simulink model "D53_LKA_Software"  (R2018b)
settings: Solver=ode3  StartTime=0.0  StopTime=10.0  FixedStep=0.01  RelTol=1e-3  EnableMultiTasking=on
model workspace (MAT data in the model file):
  MCOS : class17 (value not decoded)
  MCOS : class17 (value not decoded)
  MCOS : class17 (value not decoded)
  MCOS : class17 (value not decoded)
  MCOS : class17 (value not decoded)
  MCOS : class17 (value not decoded)
  MCOS : class17 (value not decoded)
  MCOS : class17 (value not decoded)
  MCOS : class17 (value not decoded)
  MCOS : class17 (value not decoded)
  MCOS : class17 (value not decoded)
  MCOS : class17 (value not decoded)
  MCOS : class17 (value not decoded)
  MCOS : class17 (value not decoded)
  MCOS : class17 (value not decoded)
  MCOS : class17 (value not decoded)
  MCOS : class17 (value not decoded)
  MCOS : class17 (value not decoded)
  MCOS : class17 (value not decoded)
  MCOS : class17 (value not decoded)
  MCOS : class17 (value not decoded)
  MCOS : class17 (value not decoded)
  MCOS : class17 (value not decoded)
  MCOS : class17 (value not decoded)
  MCOS : class17 (value not decoded)
  MCOS : class17 (value not decoded)
  MCOS : class17 (value not decoded)
  MCOS : class17 (value not decoded)
  MCOS : class17 (value not decoded)
  MCOS : class17 (value not decoded)
  MCOS : class17 (value not decoded)
  MCOS : class17 (value not decoded)
  MCOS : class17 (value not decoded)
  MCOS : class17 (value not decoded)
  MCOS : class17 (value not decoded)
  MCOS : class17 (value not decoded)
  MCOS : class17 (value not decoded)
  MCOS : class17 (value not decoded)
  MCOS : class17 (value not decoded)
  MCOS : class17 (value not decoded)
  MCOS : class17 (value not decoded)
  MCOS : class17 (value not decoded)
  MCOS : class17 (value not decoded)
  MCOS : class17 (value not decoded)
  MCOS : class17 (value not decoded)
  MCOS : class17 (value not decoded)
  MCOS : class17 (value not decoded)
  MCOS : class17 (value not decoded)
  MCOS : class17 (value not decoded)
  MCOS : class17 (value not decoded)
  MCOS : class17 (value not decoded)
  MCOS : class17 (value not decoded)
  MCOS : class17 (value not decoded)
  MCOS : class17 (value not decoded)
  MCOS : class17 (value not decoded)
  MCOS : class17 (value not decoded)
  MCOS : class17 (value not decoded)
  MCOS : class17 (value not decoded)
  MCOS : class17 (value not decoded)
  MCOS : class17 (value not decoded)
  MCOS : class17 (value not decoded)
  MCOS : class17 (value not decoded)
  MCOS : class17 (value not decoded)
  MCOS : class17 (value not decoded)
  MCOS : class17 (value not decoded)
  MCOS : class17 (value not decoded)
  MCOS : class17 (value not decoded)
  MCOS : class17 (value not decoded)
  MCOS : class17 (value not decoded)
  MCOS : class17 (value not decoded)
  MCOS : class17 (value not decoded)
  MCOS : class17 (value not decoded)
  MCOS : class17 (value not decoded)
  MCOS : class17 (value not decoded)
  MCOS : class17 (value not decoded)
  MCOS : class17 (value not decoded)
  MCOS : class17 (value not decoded)
  MCOS : class17 (value not decoded)
  MCOS : class17 (value not decoded)
  MCOS : class17 (value not decoded)
  MCOS : class17 (value not decoded)
  MCOS : class17 (value not decoded)
  MCOS : class17 (value not decoded)
  MCOS : class17 (value not decoded)
  MCOS : class17 (value not decoded)
  MCOS : class17 (value not decoded)
  MCOS : class17 (value not decoded)
  MCOS : class17 (value not decoded)
  MCOS : class17 (value not decoded)
undefined symbols (not defined in the file or in its folder): LKA_CarWidth, LKA_SampleTime, LKA_StrRatio_C, LKA_Veh2CamL_C, LKA_Veh2CamW_C, LKA_WhlBaseL_C, LL_CompSWA_C, LL_CrvtPrvwT_C, LL_DesDvt_C, LL_DvtComp_C, LL_DvtPrvwT_C, LL_DvtSpdDet_vDvtSpdMin_C, LL_HdAgExT_C, LL_HdAgPrvwT_C, LL_LAccMax_C, LL_LAccRMax_C, LL_LDW_EarliestWarnLine_C, LL_LDW_LatestWarnLine_C, LL_LDWS_SUPPRESS_HEADING, LL_LFClb_TFC_DiffCtlBalance, LL_LFClb_TFC_DiffCtrlMaxSWA, LL_LFClb_TFC_DiffCtrlRatio, LL_LFClb_TFC_facmGainLutGain1_C, LL_LFClb_TFC_facmGainLutGain2_C, LL_LFClb_TFC_facmIntegRatio, LL_LFClb_TFC_facmKlat_C, LL_LFClb_TFC_FfCtlRatio_C, LL_LFClb_TFC_phiIntegCtlMaxSWA_C, LL_LFClb_TFC_tiKlatPrvwT_C, LL_LFClb_TFC_vGainLutVehSpdLwr_C, LL_LFClb_TFC_vGainLutVehSpdUpr_C, LL_LKA_EarliestWarnLine_C, LL_LKA_LatestWarnLine_C, LL_LKAExPrcs_ExitC0Dvt, LL_LKAExPrcs_ExitC0Swt, LL_LKAExPrcs_tiExitTime1, LL_LKAExPrcs_tiExitTime2, LL_LKAExPrcs_tiExitTime3, LL_LKAS_OUT_OF_CONTROL_LAT_VEL, LL_LKAS_OUT_OF_CONTROL_TTLC, LL_LKASWASyn_M0, LL_LKASWASyn_M1, LL_LKASWASyn_M2, LL_LKASWASyn_M3K, LL_LKASWASyn_SWAaddMax, LL_LKASWASyn_T2, LL_LKASWASyn_tiTrqSwaRtTime, LL_LKASWASyn_tiTrqSwaTime, LL_LKASWASyn_TrqMax, LL_LKASWASyn_TrqSwaAddSwt, LL_LKASWASyn_TrqSwaRateDiff, LL_LSpdCompT_C, LL_lStpLngth_C, LL_MAX_DELAY_EPSSTAR_TIME, LL_MAX_DRIVER_TORQUE_DISABLE, LL_MAX_DRIVER_TORQUE_ENABLE, LL_MAX_LANE_WIDTH_DISABLE, LL_MAX_LANE_WIDTH_ENABLE, LL_MAX_LAT_ACC_DISABLE, LL_MAX_LAT_ACC_ENABLE ... (+30)
libraries: simulink x167, canmsglib x52, dspstat3 x3, simulink_extras x1
(part 5 of 21)

== system D53_LKA_Software/LLClb_bsLLClb_Read_Num=100/Subsystem2 ==
  In1 : Inport
  In2 : Inport  Port=2
  Data Type Conversion{1..10} (10 alike) : DataTypeConversion  OutDataTypeStr=single
  If1 : If  IfExpression=u1 ==1  ElseIfExpressions=u1==2,u1==3,u1==4,u1==5,u1==6,u1==7,u1==8,u1==9,u1==10  ShowElse=off
  Rate Transition{1..3,5..11} (10 alike) : RateTransition  Deterministic=off  OutPortSampleTime=0.01
  Subsystem2 : Subsystem
  Out1 : Outport
  Out2 : Outport  Port=2
  Out3 : Outport  Port=3
  Out4 : Outport  Port=4
  Out5 : Outport  Port=5
  Out6 : Outport  Port=6
  Out7 : Outport  Port=7
  Out8 : Outport  Port=8
  Out9 : Outport  Port=9
  Out10 : Outport  Port=10
  wires:
  Subsystem2/10(Out10) -> Data Type Conversion10/1
  Subsystem2/4(Out4) -> Data Type Conversion4/1
  If1/3 -> Subsystem2/3(In3)
  Subsystem2/7(Out7) -> Data Type Conversion7/1
  Subsystem2/1(Out1) -> Data Type Conversion1/1
  Subsystem2/9(Out9) -> Data Type Conversion9/1
  If1/6 -> Subsystem2/6(In6)
  If1/2 -> Subsystem2/2(In2)
  If1/5 -> Subsystem2/5(In5)
  Subsystem2/8(Out8) -> Data Type Conversion8/1
  If1/9 -> Subsystem2/9(In9)
  If1/4 -> Subsystem2/4(In4)
  If1/1 -> Subsystem2/1(In1)
  If1/7 -> Subsystem2/7(In7)
  If1/8 -> Subsystem2/8(In8)
  Subsystem2/3(Out3) -> Data Type Conversion3/1
  Subsystem2/2(Out2) -> Data Type Conversion2/1
  If1/10 -> Subsystem2/10(In10)
  Subsystem2/5(Out5) -> Data Type Conversion5/1
  Subsystem2/6(Out6) -> Data Type Conversion6/1
  In1/1 -> If1/1
  In2/1 -> Subsystem2/11(In11)
  Data Type Conversion1/1 -> Rate Transition1/1
  Data Type Conversion2/1 -> Rate Transition2/1
  Data Type Conversion3/1 -> Rate Transition3/1
  Data Type Conversion4/1 -> Rate Transition5/1
  Data Type Conversion5/1 -> Rate Transition6/1
  Data Type Conversion6/1 -> Rate Transition7/1
  Data Type Conversion7/1 -> Rate Transition8/1
  Data Type Conversion8/1 -> Rate Transition9/1
  Data Type Conversion9/1 -> Rate Transition10/1
  Data Type Conversion10/1 -> Rate Transition11/1
  Rate Transition1/1 -> Out1/1
  Rate Transition2/1 -> Out2/1
  Rate Transition3/1 -> Out3/1
  Rate Transition5/1 -> Out4/1
  Rate Transition6/1 -> Out5/1
  Rate Transition7/1 -> Out6/1
  Rate Transition8/1 -> Out7/1
  Rate Transition9/1 -> Out8/1
  Rate Transition10/1 -> Out9/1
  Rate Transition11/1 -> Out10/1

== system D53_LKA_Software/LLClb_bsLLClb_Read_Num=100/Subsystem3 ==
  In1 : Inport
  In2 : Inport  Port=2
  Data Type Conversion{1..10} (10 alike) : DataTypeConversion  OutDataTypeStr=single
  If1 : If  IfExpression=u1 ==11  ElseIfExpressions=u1==12,u1==13,u1==14,u1==15,u1==16,u1==17,u1==18,u1==19,u1==20  ShowElse=off
  Rate Transition{1..3,5..11} (10 alike) : RateTransition  Deterministic=off  OutPortSampleTime=0.01
  Subsystem2 : Subsystem
  Out1 : Outport
  Out2 : Outport  Port=2
  Out3 : Outport  Port=3
  Out4 : Outport  Port=4
  Out5 : Outport  Port=5
  Out6 : Outport  Port=6
  Out7 : Outport  Port=7
  Out8 : Outport  Port=8
  Out9 : Outport  Port=9
  Out10 : Outport  Port=10
  wires:
  If1/10 -> Subsystem2/10(In10)
  If1/8 -> Subsystem2/8(In8)
  If1/7 -> Subsystem2/7(In7)
  If1/1 -> Subsystem2/1(In1)
  If1/4 -> Subsystem2/4(In4)
  If1/9 -> Subsystem2/9(In9)
  If1/5 -> Subsystem2/5(In5)
  If1/2 -> Subsystem2/2(In2)
  If1/6 -> Subsystem2/6(In6)
  If1/3 -> Subsystem2/3(In3)
  In2/1 -> Subsystem2/11(In11)
  In1/1 -> If1/1
  Data Type Conversion3/1 -> Rate Transition3/1
  Data Type Conversion2/1 -> Rate Transition2/1
  Data Type Conversion10/1 -> Rate Transition11/1
  Data Type Conversion5/1 -> Rate Transition6/1
  Rate Transition6/1 -> Out5/1
  Subsystem2/5(Out5) -> Data Type Conversion5/1
  Subsystem2/6(Out6) -> Data Type Conversion6/1
  Subsystem2/10(Out10) -> Data Type Conversion10/1
  Subsystem2/1(Out1) -> Data Type Conversion1/1
  Subsystem2/9(Out9) -> Data Type Conversion9/1
  Subsystem2/7(Out7) -> Data Type Conversion7/1
  Subsystem2/8(Out8) -> Data Type Conversion8/1
  Subsystem2/3(Out3) -> Data Type Conversion3/1
  Subsystem2/4(Out4) -> Data Type Conversion4/1
  Data Type Conversion4/1 -> Rate Transition5/1
  Data Type Conversion8/1 -> Rate Transition9/1
  Data Type Conversion9/1 -> Rate Transition10/1
  Data Type Conversion7/1 -> Rate Transition8/1
  Rate Transition8/1 -> Out7/1
  Rate Transition1/1 -> Out1/1
  Rate Transition2/1 -> Out2/1
  Rate Transition5/1 -> Out4/1
  Rate Transition10/1 -> Out9/1
  Rate Transition11/1 -> Out10/1
  Rate Transition3/1 -> Out3/1
  Subsystem2/2(Out2) -> Data Type Conversion2/1
  Data Type Conversion6/1 -> Rate Transition7/1
  Rate Transition7/1 -> Out6/1
  Data Type Conversion1/1 -> Rate Transition1/1
  Rate Transition9/1 -> Out8/1

== system D53_LKA_Software/LLClb_bsLLClb_Read_Num=100/Subsystem4 ==
  In1 : Inport
  In2 : Inport  Port=2
  Data Type Conversion{1..10} (10 alike) : DataTypeConversion  OutDataTypeStr=single
  If1 : If  IfExpression=u1 ==21  ElseIfExpressions=u1==22,u1==23,u1==24,u1==25,u1==26,u1==27,u1==28,u1==29,u1==30  ShowElse=off
  Rate Transition{1..3,5..11} (10 alike) : RateTransition  Deterministic=off  OutPortSampleTime=0.01
  Subsystem2 : Subsystem
  Out1 : Outport
  Out2 : Outport  Port=2
  Out3 : Outport  Port=3
  Out4 : Outport  Port=4
  Out5 : Outport  Port=5
  Out6 : Outport  Port=6
  Out7 : Outport  Port=7
  Out8 : Outport  Port=8
  Out9 : Outport  Port=9
  Out10 : Outport  Port=10
  wires:
  If1/3 -> Subsystem2/3(In3)
  If1/6 -> Subsystem2/6(In6)
  If1/2 -> Subsystem2/2(In2)
  If1/5 -> Subsystem2/5(In5)
  If1/9 -> Subsystem2/9(In9)
  If1/4 -> Subsystem2/4(In4)
  If1/1 -> Subsystem2/1(In1)
  If1/7 -> Subsystem2/7(In7)
  If1/8 -> Subsystem2/8(In8)
  If1/10 -> Subsystem2/10(In10)
  In1/1 -> If1/1
  In2/1 -> Subsystem2/11(In11)
  Data Type Conversion3/1 -> Rate Transition3/1
  Data Type Conversion2/1 -> Rate Transition2/1
  Data Type Conversion10/1 -> Rate Transition11/1
  Data Type Conversion5/1 -> Rate Transition6/1
  Rate Transition6/1 -> Out5/1
  Subsystem2/5(Out5) -> Data Type Conversion5/1
  Subsystem2/6(Out6) -> Data Type Conversion6/1
  Subsystem2/10(Out10) -> Data Type Conversion10/1
  Subsystem2/1(Out1) -> Data Type Conversion1/1
  Subsystem2/9(Out9) -> Data Type Conversion9/1
  Subsystem2/7(Out7) -> Data Type Conversion7/1
  Subsystem2/8(Out8) -> Data Type Conversion8/1
  Subsystem2/3(Out3) -> Data Type Conversion3/1
  Subsystem2/4(Out4) -> Data Type Conversion4/1
  Data Type Conversion4/1 -> Rate Transition5/1
  Data Type Conversion8/1 -> Rate Transition9/1
  Data Type Conversion9/1 -> Rate Transition10/1
  Data Type Conversion7/1 -> Rate Transition8/1
  Rate Transition8/1 -> Out7/1
  Rate Transition1/1 -> Out1/1
  Rate Transition2/1 -> Out2/1
  Rate Transition5/1 -> Out4/1
  Rate Transition10/1 -> Out9/1
  Rate Transition11/1 -> Out10/1
  Rate Transition3/1 -> Out3/1
  Subsystem2/2(Out2) -> Data Type Conversion2/1
  Data Type Conversion6/1 -> Rate Transition7/1
  Rate Transition7/1 -> Out6/1
  Data Type Conversion1/1 -> Rate Transition1/1
  Rate Transition9/1 -> Out8/1

== system D53_LKA_Software/LLClb_bsLLClb_Read_Num=100/Subsystem5 ==
  In1 : Inport
  In2 : Inport  Port=2
  Constant : Constant  Value=10
  Data Type Conversion1 : DataTypeConversion  OutDataTypeStr=single
  Data Type Conversion3 : DataTypeConversion  OutDataTypeStr=single
  Divide : Product  Inputs=**
  Fcn : Fcn  Expr=pow(u(1),u(2))
  Mux : Mux  Inputs=2
  Out1 : Outport
  wires:
  Mux/1 -> Fcn/1
  Fcn/1 -> Divide/1
  In2/1 -> Divide/2
  Divide/1 -> Out1/1
  In1/1 -> Data Type Conversion1/1
  Data Type Conversion1/1 -> Mux/2
  Data Type Conversion3/1 -> Mux/1
  Constant/1 -> Data Type Conversion3/1

== system D53_LKA_Software/Resource Initialization/CAN Setup ==
  S-Function : S-Function  FunctionName=CAN_Init_D  Parameters=uint8(Device_Index-1),uint8(CAN0_En),uint8(CAN0_Baudrate-1),uint8(CAN1_En),uint8(CAN1_Baudrate-1),uint8(CAN2_En),uint8(CAN2_Baudrate-1),uint8(CAN3_En),uint8(CAN3_Baudrate-1)  SFunctionDeploymentMode=off  EnableBusSupport=off

== system D53_LKA_Software/Resource Initialization/DI ==

== system D53_LKA_Software/Resource Initialization/DO ==

== system D53_LKA_Software/Resource Initialization/SPI ==

== system D53_LKA_Software/Signal Output and Processing (DACOut)/D53_EPS_Control_LKA ==
  LKA_STATE_in : Inport
  LXA_ACTIVATION_in : Inport  Port=2
  LKA_TRQ_FACT_REQ_in : Inport  Port=3
  COLUMN_ANGLE_SETPOINT_in : Inport  Port=4
  Constant{2..9} (8 alike) : Constant  Value=0  OutDataTypeStr=single
  Data Type Conversion : DataTypeConversion  OutDataTypeStr=single
  DMD_DELEST_ABS_ESP : Outport
  REQ_DECON_ASR : Outport  Port=2
  LKA_TRQ_FACT_REQ : Outport  Port=3
  COLUMN_ANGLE_SETPOINT : Outport  Port=4
  ACPK_VAL_REQUEST_BSI : Outport  Port=5
  DMD_DELEST_EASYMOVE : Outport  Port=6
  LKA_STATE : Outport  Port=7
  LXA_ACTIVATION : Outport  Port=8
  DMD_DELEST_DA : Outport  Port=9
  TRAILER_DETECTION : Outport  Port=10
  CPT_PROCESS : Outport  Port=11
  CHKSUM_TRME : Outport  Port=12
  wires:
  LKA_STATE_in/1 -> Data Type Conversion/1
  Data Type Conversion/1 -> LKA_STATE/1
  COLUMN_ANGLE_SETPOINT_in/1 -> COLUMN_ANGLE_SETPOINT/1
  Constant2/1 -> DMD_DELEST_DA/1
  LXA_ACTIVATION_in/1 -> LXA_ACTIVATION/1
  LKA_TRQ_FACT_REQ_in/1 -> LKA_TRQ_FACT_REQ/1
  Constant3/1 -> TRAILER_DETECTION/1
  Constant4/1 -> DMD_DELEST_EASYMOVE/1
  Constant5/1 -> DMD_DELEST_ABS_ESP/1
  Constant6/1 -> CHKSUM_TRME/1
  Constant7/1 -> CPT_PROCESS/1
  Constant8/1 -> REQ_DECON_ASR/1
  Constant9/1 -> ACPK_VAL_REQUEST_BSI/1

== system D53_LKA_Software/Signal Output and Processing (DACOut)/D53_HMI_Control_LKA ==
  LL_bsLLHMI : Inport
  Bus Selector3 : BusSelector  OutputSignals=Hands_off_warning,HMI_Popup_Status,LDW_Flag,LDW_Status_Display,LKA_action_indication,LKA_Status_Display,Vehicle_Lane_Display
  Constant{,1..7} (8 alike) : Constant  Value=0  OutDataTypeStr=uint16
  ECU_operating_phase : Outport
  HMI_Popup_Status : Outport  Port=2
  Hands_off_warning : Outport  Port=3
  ISA_Popup_text : Outport  Port=4
  ISA_Sign_Type : Outport  Port=5
  ISA_Status : Outport  Port=6
  ISA_Value : Outport  Port=7
  LDW_Flag : Outport  Port=8
  LDW_Status_Display : Outport  Port=9
  LKA_Mode_from_Camera : Outport  Port=10
  LKA_Status_Display : Outport  Port=11
  LKA_Switch_State : Outport  Port=12
  LKA_action_indication : Outport  Port=13
  TSR_Vision_Only_Sign_Type : Outport  Port=14
  Vehicle_Lane_Display : Outport  Port=15
  wires:
  Bus Selector3/1 -> Hands_off_warning/1  "<Hands_off_warning>"
  Bus Selector3/3 -> LDW_Flag/1  "<LDW_Flag>"
  Bus Selector3/4 -> LDW_Status_Display/1  "<LDW_Status_Display>"
  Bus Selector3/5 -> LKA_action_indication/1  "<LKA_action_indication>"
  Bus Selector3/6 -> LKA_Status_Display/1  "<LKA_Status_Display>"
  Bus Selector3/7 -> Vehicle_Lane_Display/1  "<Vehicle_Lane_Display>"
  Bus Selector3/2 -> HMI_Popup_Status/1  "<HMI_Popup_Status>"
  LL_bsLLHMI/1 -> Bus Selector3/1
  Constant/1 -> ECU_operating_phase/1
  Constant1/1 -> ISA_Popup_text/1
  Constant2/1 -> ISA_Sign_Type/1
  Constant4/1 -> ISA_Value/1
  Constant3/1 -> ISA_Status/1
  Constant5/1 -> LKA_Mode_from_Camera/1
  Constant6/1 -> LKA_Switch_State/1
  Constant7/1 -> TSR_Vision_Only_Sign_Type/1

== system D53_LKA_Software/SignalBusCreator/Body Electric System State Receive and Processing (BESRx) ==
  Bus Creator1 : BusCreator  Inputs=11
  Steering Lamp CAN Frame PreProcess (StLampCANFrmPPrcs) : Subsystem
  bsDoorsState : Constant  Value=0  OutDataTypeStr=uint16
  bsWiperState : Constant  Value=0  OutDataTypeStr=uint16
  BESRx_bsBESState : Outport
  wires:
  Steering Lamp CAN Frame PreProcess (StLampCANFrmPPrcs)/9(Out9) -> Bus Creator1/11  "MP5_AEB_Activation_Config"
  bsWiperState/1 -> Bus Creator1/3  "bsWiperState"
  bsDoorsState/1 -> Bus Creator1/2  "bsDoorsState"
  Bus Creator1/1 -> BESRx_bsBESState/1
  Steering Lamp CAN Frame PreProcess (StLampCANFrmPPrcs)/6(Out6) -> Bus Creator1/8  "IC_FCW_Sensitivity"
  Steering Lamp CAN Frame PreProcess (StLampCANFrmPPrcs)/5(Out5) -> Bus Creator1/7  "GW_BCM_Brakeonly_Request_BCM"
  Steering Lamp CAN Frame PreProcess (StLampCANFrmPPrcs)/3(Out3) -> Bus Creator1/6  "BCM_State_Front_Wiper"
  Steering Lamp CAN Frame PreProcess (StLampCANFrmPPrcs)/2(Out2) -> Bus Creator1/5  "BCM_CHMSLStatus"
  Steering Lamp CAN Frame PreProcess (StLampCANFrmPPrcs)/1(Out1) -> Bus Creator1/4  "BCM_BrakeLampStatu"
  Steering Lamp CAN Frame PreProcess (StLampCANFrmPPrcs)/4(CANFrmPPrcs_stLStLamp) -> Bus Creator1/1  "StrLampRx_bsStrLampState"
  Steering Lamp CAN Frame PreProcess (StLampCANFrmPPrcs)/7(Out7) -> Bus Creator1/9  "IC_Fcw_Activation_Config"
  Steering Lamp CAN Frame PreProcess (StLampCANFrmPPrcs)/8(Out8) -> Bus Creator1/10  "IC_seat_bealt_passenger_state"

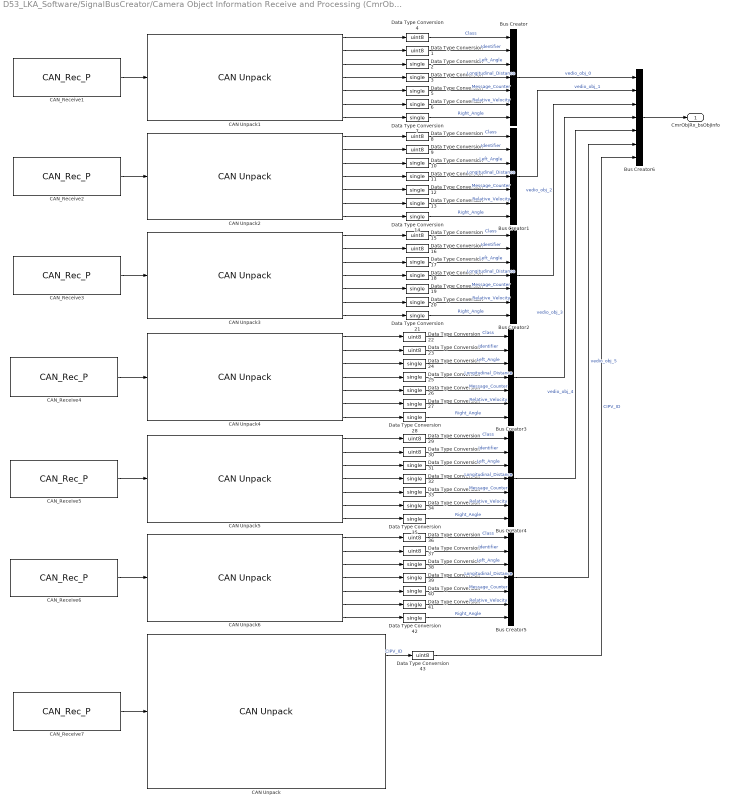
== system D53_LKA_Software/SignalBusCreator/Camera Object Information Receive and Processing (CmrObjRx) ==
  Bus Creator{,1..6} (7 alike) : BusCreator  Inputs=7
  CAN Unpack : canmsglib/CAN Unpack  CANdbFile=F:\ADAS_File\ACC_AEB_D53_20190520\ADAS_ECU_S_CAN_V2_v20190314.dbc  MsgList=Video_Object_Header  MsgName=Video_Object_Header  MsgIDType=Standard (11-bit identifier)  MsgIdentifier=1078  MsgLength=6  SignalInfo=AEB_Availability$0$1$2$2$1$0$1$0$0$1$#CIPV_FCV$9$2$2$2$1$0$1$0$0$3$#CIPV_ID$25$7$2$2$1$0$1$0$0$127$#Left_Close_Range_Cut_In$2$1$2$2$1$0$1$0$0$1$#MCPB_FCV$46$2$2$2$1$0$1$0$0$3$#MCPB_ID$33$7$2$2$1$0$1$0$0$127$#Message_Counter$22$2$2$2$1$0$1$0$0$3$#Number_Of_Objects$3$5$2$2$1$0$1$0$0$31$#PED_CYC_ABA_ALERT$17$1$2$2$1$0$1$0$0$1$#PED_CYC_AEB_ALERT$16$1$2$2$1$0$1$0$0$1$#PED_CYC_DANGER_ZONE$20$2$2$2$1$0$1$0$0$3$#PED_CYC_FCW_ALERT$19$1$2$2$1$0$1$0$0$1$#PED_CYC_PREFILL_ALERT$18$1$2$2$1$0$1$0$0$1$#Right_Close_Range_Cut_In$1$1$2$2$1$0$1$0$0$1$#VEH_ABA_ALERT$13$1$2$2$1$0$1$0$0$1$#VEH_AEB_ALERT$12$1$2$2$1$0$1$0$0$1$#VEH_FCW_ALERT$15$1$2$2$1$0$1$0$0$1$#VEH_PREFILL_ALERT$14$1$2$2$1$0$1$0$0$1$#VEH_RESERVED_ALERT$11$1$2$2$1$0$1$0$0$1$#  NSignals=19  IDPort=off  TimestampPort=off  ErrorPort=off  RemotePort=off  LengthPort=off  StatusPort=off  StartBits=str2num('[int32(0);int32(9);int32(25);int32(2);int32(46);int32(33);int32(22);int32(3);int32(17);int32(16);int32(20);int32(19);int32(18);int32(1);int32(13);int32(12);int32(15);int32(14);int32(11)]')  SignalSizes=str2num('[int32(1);int32(2);int32(7);int32(1);int32(2);int32(7);int32(2);int32(5);int32(1);int32(1);int32(2);int32(1);int32(1);int32(1);int32(1);int32(1);int32(1);int32(1);int32(1)]')  ByteOrders=str2num('[int32(2);int32(2);int32(2);int32(2);int32(2);int32(2);int32(2);int32(2);int32(2);int32(2);int32(2);int32(2);int32(2);int32(2);int32(2);int32(2);int32(2);int32(2);int32(2)]')  DataTypes=str2num('[int32(2);int32(2);int32(2);int32(2);int32(2);int32(2);int32(2);int32(2);int32(2);int32(2);int32(2);int32(2);int32(2);int32(2);int32(2);int32(2);int32(2);int32(2);int32(2)]')  MultiplexTypes=str2num('[int32(1);int32(1);int32(1);int32(1);int32(1);int32(1);int32(1);int32(1);int32(1);int32(1);int32(1);int32(1);int32(1);int32(1);int32(1);int32(1);int32(1);int32(1);int32(1)]')  MultiplexValues=str2num('[double(0);double(0);double(0);double(0);double(0);double(0);double(0);double(0);double(0);double(0);double(0);double(0);double(0);double(0);double(0);double(0);double(0);double(0);double(0)]')  Factors=str2num('[double(1);double(1);double(1);double(1);double(1);double(1);double(1);double(1);double(1);double(1);double(1);double(1);double(1);double(1);double(1);double(1);double(1);double(1);double(1)]')  Offsets=str2num('[double(0);double(0);double(0);double(0);double(0);double(0);double(0);double(0);double(0);double(0);double(0);double(0);double(0);double(0);double(0);double(0);double(0);double(0);double(0)]')  Minimums=str2num('[double(0);double(0);double(0);double(0);double(0);double(0);double(0);double(0);double(0);double(0);double(0);double(0);double(0);double(0);double(0);double(0);double(0);double(0);double(0)]')  Maximums=str2num('[double(1);double(3);double(127);double(1);double(3);double(127);double(3);double(31);double(1);double(1);double(3);double(1);double(1);double(1);double(1);double(1);double(1);double(1);double(1)]')  ApplyMinMax=off
      settings: SourceProductName=Simulink Real-Time  SourceProductBaseCode=XP  DataFormat=CANdb specified signals
  CAN Unpack1 : canmsglib/CAN Unpack  CANdbFile=F:\ADAS_File\ACC_AEB_D53_20190520\ADAS_ECU_S_CAN_V2_v20190314.dbc  MsgList=Video_Object_0_A  MsgName=Video_Object_0_A  MsgIDType=Standard (11-bit identifier)  MsgIdentifier=1792  MsgLength=8  SignalInfo=Class_700$56$3$2$2$1$0$1$0$0$7$#Identifier_700$1$7$2$2$1$0$1$0$0$127$#Left_Angle_700$41$13$2$1$1$0$2.000000e-04$0$-8.192000e-01$8.190000e-01$#Longitudinal_Distance_700$20$12$2$2$1$0$5.000000e-02$0$0$2.047500e+02$#Message_Counter_700$38$2$2$2$1$0$1$0$0$3$#Relative_Velocity_700$24$12$2$1$1$0$5.000000e-02$0$-1.024000e+02$1.023500e+02$#Right_Angle_700$59$13$2$1$1$0$2.000000e-04$0$-8.192000e-01$8.190000e-01$#  NSignals=7  IDPort=off  TimestampPort=off  ErrorPort=off  RemotePort=off  LengthPort=off  StatusPort=off  StartBits=str2num('[int32(56);int32(1);int32(41);int32(20);int32(38);int32(24);int32(59)]')  SignalSizes=str2num('[int32(3);int32(7);int32(13);int32(12);int32(2);int32(12);int32(13)]')  ByteOrders=str2num('[int32(2);int32(2);int32(2);int32(2);int32(2);int32(2);int32(2)]')  DataTypes=str2num('[int32(2);int32(2);int32(1);int32(2);int32(2);int32(1);int32(1)]')  MultiplexTypes=str2num('[int32(1);int32(1);int32(1);int32(1);int32(1);int32(1);int32(1)]')  MultiplexValues=str2num('[double(0);double(0);double(0);double(0);double(0);double(0);double(0)]')  Factors=str2num('[double(1);double(1);double(2.000000e-04);double(5.000000e-02);double(1);double(5.000000e-02);double(2.000000e-04)]')  Offsets=str2num('[double(0);double(0);double(0);double(0);double(0);double(0);double(0)]')  Minimums=str2num('[double(0);double(0);double(-8.192000e-01);double(0);double(0);double(-1.024000e+02);double(-8.192000e-01)]')  Maximums=str2num('[double(7);double(127);double(8.190000e-01);double(2.047500e+02);double(3);double(1.023500e+02);double(8.190000e-01)]')  ApplyMinMax=off
      settings: SourceProductName=Simulink Real-Time  SourceProductBaseCode=XP  DataFormat=CANdb specified signals
  CAN Unpack2 : canmsglib/CAN Unpack  CANdbFile=F:\ADAS_File\ACC_AEB_D53_20190520\ADAS_ECU_S_CAN_V2_v20190314.dbc  MsgList=Video_Object_1_A  MsgName=Video_Object_1_A  MsgIDType=Standard (11-bit identifier)  MsgIdentifier=1796  MsgLength=8  SignalInfo=Class_704$56$3$2$2$1$0$1$0$0$7$#Identifier_704$1$7$2$2$1$0$1$0$0$127$#Left_Angle_704$41$13$2$1$1$0$2.000000e-04$0$-8.192000e-01$8.190000e-01$#Longitudinal_Distance_704$20$12$2$2$1$0$5.000000e-02$0$0$2.047500e+02$#Message_Counter_704$38$2$2$2$1$0$1$0$0$3$#Relative_Velocity_704$24$12$2$1$1$0$5.000000e-02$0$-1.024000e+02$1.023500e+02$#Right_Angle_704$59$13$2$1$1$0$2.000000e-04$0$-8.192000e-01$8.190000e-01$#  NSignals=7  IDPort=off  TimestampPort=off  ErrorPort=off  RemotePort=off  LengthPort=off  StatusPort=off  StartBits=str2num('[int32(56);int32(1);int32(41);int32(20);int32(38);int32(24);int32(59)]')  SignalSizes=str2num('[int32(3);int32(7);int32(13);int32(12);int32(2);int32(12);int32(13)]')  ByteOrders=str2num('[int32(2);int32(2);int32(2);int32(2);int32(2);int32(2);int32(2)]')  DataTypes=str2num('[int32(2);int32(2);int32(1);int32(2);int32(2);int32(1);int32(1)]')  MultiplexTypes=str2num('[int32(1);int32(1);int32(1);int32(1);int32(1);int32(1);int32(1)]')  MultiplexValues=str2num('[double(0);double(0);double(0);double(0);double(0);double(0);double(0)]')  Factors=str2num('[double(1);double(1);double(2.000000e-04);double(5.000000e-02);double(1);double(5.000000e-02);double(2.000000e-04)]')  Offsets=str2num('[double(0);double(0);double(0);double(0);double(0);double(0);double(0)]')  Minimums=str2num('[double(0);double(0);double(-8.192000e-01);double(0);double(0);double(-1.024000e+02);double(-8.192000e-01)]')  Maximums=str2num('[double(7);double(127);double(8.190000e-01);double(2.047500e+02);double(3);double(1.023500e+02);double(8.190000e-01)]')  ApplyMinMax=off
      settings: SourceProductName=Simulink Real-Time  SourceProductBaseCode=XP  DataFormat=CANdb specified signals
  CAN Unpack3 : canmsglib/CAN Unpack  CANdbFile=F:\ADAS_File\ACC_AEB_D53_20190520\ADAS_ECU_S_CAN_V2_v20190314.dbc  MsgList=Video_Object_2_A  MsgName=Video_Object_2_A  MsgIDType=Standard (11-bit identifier)  MsgIdentifier=1800  MsgLength=8  SignalInfo=Class_708$56$3$2$2$1$0$1$0$0$7$#Identifier_708$1$7$2$2$1$0$1$0$0$127$#Left_Angle_708$41$13$2$1$1$0$2.000000e-04$0$-8.192000e-01$8.190000e-01$#Longitudinal_Distance_708$20$12$2$2$1$0$5.000000e-02$0$0$2.047500e+02$#Message_Counter_708$38$2$2$2$1$0$1$0$0$3$#Relative_Velocity_708$24$12$2$1$1$0$5.000000e-02$0$-1.024000e+02$1.023500e+02$#Right_Angle_708$59$13$2$1$1$0$2.000000e-04$0$-8.192000e-01$8.190000e-01$#  NSignals=7  IDPort=off  TimestampPort=off  ErrorPort=off  RemotePort=off  LengthPort=off  StatusPort=off  StartBits=str2num('[int32(56);int32(1);int32(41);int32(20);int32(38);int32(24);int32(59)]')  SignalSizes=str2num('[int32(3);int32(7);int32(13);int32(12);int32(2);int32(12);int32(13)]')  ByteOrders=str2num('[int32(2);int32(2);int32(2);int32(2);int32(2);int32(2);int32(2)]')  DataTypes=str2num('[int32(2);int32(2);int32(1);int32(2);int32(2);int32(1);int32(1)]')  MultiplexTypes=str2num('[int32(1);int32(1);int32(1);int32(1);int32(1);int32(1);int32(1)]')  MultiplexValues=str2num('[double(0);double(0);double(0);double(0);double(0);double(0);double(0)]')  Factors=str2num('[double(1);double(1);double(2.000000e-04);double(5.000000e-02);double(1);double(5.000000e-02);double(2.000000e-04)]')  Offsets=str2num('[double(0);double(0);double(0);double(0);double(0);double(0);double(0)]')  Minimums=str2num('[double(0);double(0);double(-8.192000e-01);double(0);double(0);double(-1.024000e+02);double(-8.192000e-01)]')  Maximums=str2num('[double(7);double(127);double(8.190000e-01);double(2.047500e+02);double(3);double(1.023500e+02);double(8.190000e-01)]')  ApplyMinMax=off
      settings: SourceProductName=Simulink Real-Time  SourceProductBaseCode=XP  DataFormat=CANdb specified signals
  CAN Unpack4 : canmsglib/CAN Unpack  CANdbFile=F:\ADAS_File\ACC_AEB_D53_20190520\ADAS_ECU_S_CAN_V2_v20190314.dbc  MsgList=Video_Object_3_A  MsgName=Video_Object_3_A  MsgIDType=Standard (11-bit identifier)  MsgIdentifier=1804  MsgLength=8  SignalInfo=Class_70C$56$3$2$2$1$0$1$0$0$7$#Identifier_70C$1$7$2$2$1$0$1$0$0$127$#Left_Angle_70C$41$13$2$1$1$0$2.000000e-04$0$-8.192000e-01$8.190000e-01$#Longitudinal_Distance_70C$20$12$2$2$1$0$5.000000e-02$0$0$2.047500e+02$#Message_Counter_70C$38$2$2$2$1$0$1$0$0$3$#Relative_Velocity_70C$24$12$2$1$1$0$5.000000e-02$0$-1.024000e+02$1.023500e+02$#Right_Angle_70C$59$13$2$1$1$0$2.000000e-04$0$-8.192000e-01$8.190000e-01$#  NSignals=7  IDPort=off  TimestampPort=off  ErrorPort=off  RemotePort=off  LengthPort=off  StatusPort=off  StartBits=str2num('[int32(56);int32(1);int32(41);int32(20);int32(38);int32(24);int32(59)]')  SignalSizes=str2num('[int32(3);int32(7);int32(13);int32(12);int32(2);int32(12);int32(13)]')  ByteOrders=str2num('[int32(2);int32(2);int32(2);int32(2);int32(2);int32(2);int32(2)]')  DataTypes=str2num('[int32(2);int32(2);int32(1);int32(2);int32(2);int32(1);int32(1)]')  MultiplexTypes=str2num('[int32(1);int32(1);int32(1);int32(1);int32(1);int32(1);int32(1)]')  MultiplexValues=str2num('[double(0);double(0);double(0);double(0);double(0);double(0);double(0)]')  Factors=str2num('[double(1);double(1);double(2.000000e-04);double(5.000000e-02);double(1);double(5.000000e-02);double(2.000000e-04)]')  Offsets=str2num('[double(0);double(0);double(0);double(0);double(0);double(0);double(0)]')  Minimums=str2num('[double(0);double(0);double(-8.192000e-01);double(0);double(0);double(-1.024000e+02);double(-8.192000e-01)]')  Maximums=str2num('[double(7);double(127);double(8.190000e-01);double(2.047500e+02);double(3);double(1.023500e+02);double(8.190000e-01)]')  ApplyMinMax=off
      settings: SourceProductName=Simulink Real-Time  SourceProductBaseCode=XP  DataFormat=CANdb specified signals
  CAN Unpack5 : canmsglib/CAN Unpack  CANdbFile=F:\ADAS_File\ACC_AEB_D53_20190520\ADAS_ECU_S_CAN_V2_v20190314.dbc  MsgList=Video_Object_4_A  MsgName=Video_Object_4_A  MsgIDType=Standard (11-bit identifier)  MsgIdentifier=1808  MsgLength=8  SignalInfo=Class_710$56$3$2$2$1$0$1$0$0$7$#Identifier_710$1$7$2$2$1$0$1$0$0$127$#Left_Angle_710$41$13$2$1$1$0$2.000000e-04$0$-8.192000e-01$8.190000e-01$#Longitudinal_Distance_710$20$12$2$2$1$0$5.000000e-02$0$0$2.047500e+02$#Message_Counter_710$38$2$2$2$1$0$1$0$0$3$#Relative_Velocity_710$24$12$2$1$1$0$5.000000e-02$0$-1.024000e+02$1.023500e+02$#Right_Angle_710$59$13$2$1$1$0$2.000000e-04$0$-8.192000e-01$8.190000e-01$#  NSignals=7  IDPort=off  TimestampPort=off  ErrorPort=off  RemotePort=off  LengthPort=off  StatusPort=off  StartBits=str2num('[int32(56);int32(1);int32(41);int32(20);int32(38);int32(24);int32(59)]')  SignalSizes=str2num('[int32(3);int32(7);int32(13);int32(12);int32(2);int32(12);int32(13)]')  ByteOrders=str2num('[int32(2);int32(2);int32(2);int32(2);int32(2);int32(2);int32(2)]')  DataTypes=str2num('[int32(2);int32(2);int32(1);int32(2);int32(2);int32(1);int32(1)]')  MultiplexTypes=str2num('[int32(1);int32(1);int32(1);int32(1);int32(1);int32(1);int32(1)]')  MultiplexValues=str2num('[double(0);double(0);double(0);double(0);double(0);double(0);double(0)]')  Factors=str2num('[double(1);double(1);double(2.000000e-04);double(5.000000e-02);double(1);double(5.000000e-02);double(2.000000e-04)]')  Offsets=str2num('[double(0);double(0);double(0);double(0);double(0);double(0);double(0)]')  Minimums=str2num('[double(0);double(0);double(-8.192000e-01);double(0);double(0);double(-1.024000e+02);double(-8.192000e-01)]')  Maximums=str2num('[double(7);double(127);double(8.190000e-01);double(2.047500e+02);double(3);double(1.023500e+02);double(8.190000e-01)]')  ApplyMinMax=off
      settings: SourceProductName=Simulink Real-Time  SourceProductBaseCode=XP  DataFormat=CANdb specified signals
  CAN Unpack6 : canmsglib/CAN Unpack  CANdbFile=F:\ADAS_File\ACC_AEB_D53_20190520\ADAS_ECU_S_CAN_V2_v20190314.dbc  MsgList=Video_Object_5_A  MsgName=Video_Object_5_A  MsgIDType=Standard (11-bit identifier)  MsgIdentifier=1812  MsgLength=8  SignalInfo=Class_714$56$3$2$2$1$0$1$0$0$7$#Identifier_714$1$7$2$2$1$0$1$0$0$127$#Left_Angle_714$41$13$2$1$1$0$2.000000e-04$0$-8.192000e-01$8.190000e-01$#Longitudinal_Distance_714$20$12$2$2$1$0$5.000000e-02$0$0$2.047500e+02$#Message_Counter_714$38$2$2$2$1$0$1$0$0$3$#Relative_Velocity_714$24$12$2$1$1$0$5.000000e-02$0$-1.024000e+02$1.023500e+02$#Right_Angle_714$59$13$2$1$1$0$2.000000e-04$0$-8.192000e-01$8.190000e-01$#  NSignals=7  IDPort=off  TimestampPort=off  ErrorPort=off  RemotePort=off  LengthPort=off  StatusPort=off  StartBits=str2num('[int32(56);int32(1);int32(41);int32(20);int32(38);int32(24);int32(59)]')  SignalSizes=str2num('[int32(3);int32(7);int32(13);int32(12);int32(2);int32(12);int32(13)]')  ByteOrders=str2num('[int32(2);int32(2);int32(2);int32(2);int32(2);int32(2);int32(2)]')  DataTypes=str2num('[int32(2);int32(2);int32(1);int32(2);int32(2);int32(1);int32(1)]')  MultiplexTypes=str2num('[int32(1);int32(1);int32(1);int32(1);int32(1);int32(1);int32(1)]')  MultiplexValues=str2num('[double(0);double(0);double(0);double(0);double(0);double(0);double(0)]')  Factors=str2num('[double(1);double(1);double(2.000000e-04);double(5.000000e-02);double(1);double(5.000000e-02);double(2.000000e-04)]')  Offsets=str2num('[double(0);double(0);double(0);double(0);double(0);double(0);double(0)]')  Minimums=str2num('[double(0);double(0);double(-8.192000e-01);double(0);double(0);double(-1.024000e+02);double(-8.192000e-01)]')  Maximums=str2num('[double(7);double(127);double(8.190000e-01);double(2.047500e+02);double(3);double(1.023500e+02);double(8.190000e-01)]')  ApplyMinMax=off
      settings: SourceProductName=Simulink Real-Time  SourceProductBaseCode=XP  DataFormat=CANdb specified signals
  CAN_Receive1 : S-Function  FunctionName=CAN_Rec_P  Parameters=uint8(Module-1),uint32(ID),uint8(Frameformat-1),uint8(Newflag),uint8(FIFO),double(sampletime)  SFunctionDeploymentMode=off  EnableBusSupport=off  mask(CAN_receive){Module=CAN_2, ID=1792, Frameformat=Standard (11-bit identifier), Newflag=off, FIFO=off, sampletime=0.01}
      mask prompts: Module "CAN Port:"; ID "CAN Frame ID:"; Frameformat "CAN Frame Format:"; FIFO "Overflow flag"
      mask init:
      | maskdisplay = canrecicon(Module,ID,Frameformat,Newflag,FIFO);
      | set_param(gcb, 'MaskDisplay', maskdisplay);
      mask TypeOptions Module: CAN_0 | CAN_1 | CAN_2 | CAN_3
      mask TypeOptions Frameformat: Standard (11-bit identifier) | Extended (29-bit identifier)
      mask Display: color('blue');text(0.98,0.9,'MPC5675K','horizontalAlignment','right');color('black');text(0.5,0.6,'FlexCAN_2 Receive','horizontalAlignment','center');text(0.5,0.35,'Standard ID:1792','horizontalAlignment','center');port_label('output',1,'CAN_Msg');
  CAN_Receive2 : S-Function  FunctionName=CAN_Rec_P  Parameters=uint8(Module-1),uint32(ID),uint8(Frameformat-1),uint8(Newflag),uint8(FIFO),double(sampletime)  SFunctionDeploymentMode=off  EnableBusSupport=off  mask(CAN_receive){Module=CAN_2, ID=1796, Frameformat=Standard (11-bit identifier), Newflag=off, FIFO=off, sampletime=0.01}
      mask prompts: Module "CAN Port:"; ID "CAN Frame ID:"; Frameformat "CAN Frame Format:"; FIFO "Overflow flag"
      mask init:
      | maskdisplay = canrecicon(Module,ID,Frameformat,Newflag,FIFO);
      | set_param(gcb, 'MaskDisplay', maskdisplay);
      mask TypeOptions Module: CAN_0 | CAN_1 | CAN_2 | CAN_3
      mask TypeOptions Frameformat: Standard (11-bit identifier) | Extended (29-bit identifier)
      mask Display: color('blue');text(0.98,0.9,'MPC5675K','horizontalAlignment','right');color('black');text(0.5,0.6,'FlexCAN_2 Receive','horizontalAlignment','center');text(0.5,0.35,'Standard ID:1796','horizontalAlignment','center');port_label('output',1,'CAN_Msg');
  CAN_Receive3 : S-Function  FunctionName=CAN_Rec_P  Parameters=uint8(Module-1),uint32(ID),uint8(Frameformat-1),uint8(Newflag),uint8(FIFO),double(sampletime)  SFunctionDeploymentMode=off  EnableBusSupport=off  mask(CAN_receive){Module=CAN_2, ID=1800, Frameformat=Standard (11-bit identifier), Newflag=off, FIFO=off, sampletime=0.01}
      mask prompts: Module "CAN Port:"; ID "CAN Frame ID:"; Frameformat "CAN Frame Format:"; FIFO "Overflow flag"
      mask init:
      | maskdisplay = canrecicon(Module,ID,Frameformat,Newflag,FIFO);
      | set_param(gcb, 'MaskDisplay', maskdisplay);
      mask TypeOptions Module: CAN_0 | CAN_1 | CAN_2 | CAN_3
      mask TypeOptions Frameformat: Standard (11-bit identifier) | Extended (29-bit identifier)
      mask Display: color('blue');text(0.98,0.9,'MPC5675K','horizontalAlignment','right');color('black');text(0.5,0.6,'FlexCAN_2 Receive','horizontalAlignment','center');text(0.5,0.35,'Standard ID:1800','horizontalAlignment','center');port_label('output',1,'CAN_Msg');
  CAN_Receive4 : S-Function  FunctionName=CAN_Rec_P  Parameters=uint8(Module-1),uint32(ID),uint8(Frameformat-1),uint8(Newflag),uint8(FIFO),double(sampletime)  SFunctionDeploymentMode=off  EnableBusSupport=off  mask(CAN_receive){Module=CAN_2, ID=1804, Frameformat=Standard (11-bit identifier), Newflag=off, FIFO=off, sampletime=0.01}
      mask prompts: Module "CAN Port:"; ID "CAN Frame ID:"; Frameformat "CAN Frame Format:"; FIFO "Overflow flag"
      mask init:
      | maskdisplay = canrecicon(Module,ID,Frameformat,Newflag,FIFO);
      | set_param(gcb, 'MaskDisplay', maskdisplay);
      mask TypeOptions Module: CAN_0 | CAN_1 | CAN_2 | CAN_3
      mask TypeOptions Frameformat: Standard (11-bit identifier) | Extended (29-bit identifier)
      mask Display: color('blue');text(0.98,0.9,'MPC5675K','horizontalAlignment','right');color('black');text(0.5,0.6,'FlexCAN_2 Receive','horizontalAlignment','center');text(0.5,0.35,'Standard ID:1804','horizontalAlignment','center');port_label('output',1,'CAN_Msg');
  CAN_Receive5 : S-Function  FunctionName=CAN_Rec_P  Parameters=uint8(Module-1),uint32(ID),uint8(Frameformat-1),uint8(Newflag),uint8(FIFO),double(sampletime)  SFunctionDeploymentMode=off  EnableBusSupport=off  mask(CAN_receive){Module=CAN_2, ID=1808, Frameformat=Standard (11-bit identifier), Newflag=off, FIFO=off, sampletime=0.01}
      mask prompts: Module "CAN Port:"; ID "CAN Frame ID:"; Frameformat "CAN Frame Format:"; FIFO "Overflow flag"
      mask init:
      | maskdisplay = canrecicon(Module,ID,Frameformat,Newflag,FIFO);
      | set_param(gcb, 'MaskDisplay', maskdisplay);
      mask TypeOptions Module: CAN_0 | CAN_1 | CAN_2 | CAN_3
      mask TypeOptions Frameformat: Standard (11-bit identifier) | Extended (29-bit identifier)
      mask Display: color('blue');text(0.98,0.9,'MPC5675K','horizontalAlignment','right');color('black');text(0.5,0.6,'FlexCAN_2 Receive','horizontalAlignment','center');text(0.5,0.35,'Standard ID:1808','horizontalAlignment','center');port_label('output',1,'CAN_Msg');
  CAN_Receive6 : S-Function  FunctionName=CAN_Rec_P  Parameters=uint8(Module-1),uint32(ID),uint8(Frameformat-1),uint8(Newflag),uint8(FIFO),double(sampletime)  SFunctionDeploymentMode=off  EnableBusSupport=off  mask(CAN_receive){Module=CAN_2, ID=1812, Frameformat=Standard (11-bit identifier), Newflag=off, FIFO=off, sampletime=0.01}
      mask prompts: Module "CAN Port:"; ID "CAN Frame ID:"; Frameformat "CAN Frame Format:"; FIFO "Overflow flag"
      mask init:
      | maskdisplay = canrecicon(Module,ID,Frameformat,Newflag,FIFO);
      | set_param(gcb, 'MaskDisplay', maskdisplay);
      mask TypeOptions Module: CAN_0 | CAN_1 | CAN_2 | CAN_3
      mask TypeOptions Frameformat: Standard (11-bit identifier) | Extended (29-bit identifier)
      mask Display: color('blue');text(0.98,0.9,'MPC5675K','horizontalAlignment','right');color('black');text(0.5,0.6,'FlexCAN_2 Receive','horizontalAlignment','center');text(0.5,0.35,'Standard ID:1812','horizontalAlignment','center');port_label('output',1,'CAN_Msg');
  CAN_Receive7 : S-Function  FunctionName=CAN_Rec_P  Parameters=uint8(Module-1),uint32(ID),uint8(Frameformat-1),uint8(Newflag),uint8(FIFO),double(sampletime)  SFunctionDeploymentMode=off  EnableBusSupport=off  mask(CAN_receive){Module=CAN_2, ID=1078, Frameformat=Standard (11-bit identifier), Newflag=off, FIFO=off, sampletime=0.01}
      mask prompts: Module "CAN Port:"; ID "CAN Frame ID:"; Frameformat "CAN Frame Format:"; FIFO "Overflow flag"
      mask init:
      | maskdisplay = canrecicon(Module,ID,Frameformat,Newflag,FIFO);
      | set_param(gcb, 'MaskDisplay', maskdisplay);
      mask TypeOptions Module: CAN_0 | CAN_1 | CAN_2 | CAN_3
      mask TypeOptions Frameformat: Standard (11-bit identifier) | Extended (29-bit identifier)
      mask Display: color('blue');text(0.98,0.9,'MPC5675K','horizontalAlignment','right');color('black');text(0.5,0.6,'FlexCAN_2 Receive','horizontalAlignment','center');text(0.5,0.35,'Standard ID:1078','horizontalAlignment','center');port_label('output',1,'CAN_Msg');
  Data Type Conversion{1,4,8..9,15..16,22..23,29..30,36..37,43} (13 alike) : DataTypeConversion  OutDataTypeStr=uint8
  Data Type Conversion{2..3,5..7,10..14,17..21,24..28,31..35,38..42} (30 alike) : DataTypeConversion  OutDataTypeStr=single
  CmrObjRx_bsObjInfo : Outport
  wires:
  Bus Creator6/1 -> CmrObjRx_bsObjInfo/1
  Data Type Conversion43/1 -> Bus Creator6/7  "CIPV_ID"
  Data Type Conversion42/1 -> Bus Creator5/7  "Right_Angle"
  Data Type Conversion41/1 -> Bus Creator5/6  "Relative_Velocity"
  Data Type Conversion40/1 -> Bus Creator5/5  "Message_Counter"
  Data Type Conversion39/1 -> Bus Creator5/4  "Longitudinal_Distance"
  Data Type Conversion38/1 -> Bus Creator5/3  "Left_Angle"
  Data Type Conversion37/1 -> Bus Creator5/2  "Identifier"
  Data Type Conversion36/1 -> Bus Creator5/1  "Class"
  Data Type Conversion35/1 -> Bus Creator4/7  "Right_Angle"
  Data Type Conversion34/1 -> Bus Creator4/6  "Relative_Velocity"
  Data Type Conversion33/1 -> Bus Creator4/5  "Message_Counter"
  Data Type Conversion32/1 -> Bus Creator4/4  "Longitudinal_Distance"
  Data Type Conversion31/1 -> Bus Creator4/3  "Left_Angle"
  Data Type Conversion30/1 -> Bus Creator4/2  "Identifier"
  Data Type Conversion29/1 -> Bus Creator4/1  "Class"
  Data Type Conversion28/1 -> Bus Creator3/7  "Right_Angle"
  Data Type Conversion27/1 -> Bus Creator3/6  "Relative_Velocity"
  Data Type Conversion26/1 -> Bus Creator3/5  "Message_Counter"
  Data Type Conversion25/1 -> Bus Creator3/4  "Longitudinal_Distance"
  Data Type Conversion24/1 -> Bus Creator3/3  "Left_Angle"
  Data Type Conversion23/1 -> Bus Creator3/2  "Identifier"
  Data Type Conversion22/1 -> Bus Creator3/1  "Class"
  Data Type Conversion21/1 -> Bus Creator2/7  "Right_Angle"
  Data Type Conversion20/1 -> Bus Creator2/6  "Relative_Velocity"
  Data Type Conversion19/1 -> Bus Creator2/5  "Message_Counter"
  Data Type Conversion18/1 -> Bus Creator2/4  "Longitudinal_Distance"
  Data Type Conversion17/1 -> Bus Creator2/3  "Left_Angle"
  Data Type Conversion16/1 -> Bus Creator2/2  "Identifier"
  Data Type Conversion15/1 -> Bus Creator2/1  "Class"
  Data Type Conversion14/1 -> Bus Creator1/7  "Right_Angle"
  Data Type Conversion13/1 -> Bus Creator1/6  "Relative_Velocity"
  Data Type Conversion12/1 -> Bus Creator1/5  "Message_Counter"
  Data Type Conversion11/1 -> Bus Creator1/4  "Longitudinal_Distance"
  Data Type Conversion10/1 -> Bus Creator1/3  "Left_Angle"
  Data Type Conversion9/1 -> Bus Creator1/2  "Identifier"
  Data Type Conversion8/1 -> Bus Creator1/1  "Class"
  Data Type Conversion7/1 -> Bus Creator/7  "Right_Angle"
  Data Type Conversion6/1 -> Bus Creator/6  "Relative_Velocity"
  Data Type Conversion5/1 -> Bus Creator/5  "Message_Counter"
  Data Type Conversion3/1 -> Bus Creator/4  "Longitudinal_Distance"
  Data Type Conversion2/1 -> Bus Creator/3  "Left_Angle"
  Data Type Conversion1/1 -> Bus Creator/2  "Identifier"
  Data Type Conversion4/1 -> Bus Creator/1  "Class"
  CAN_Receive7/1 -> CAN Unpack/1
  CAN_Receive6/1 -> CAN Unpack6/1
  CAN_Receive5/1 -> CAN Unpack5/1
  CAN_Receive4/1 -> CAN Unpack4/1
  CAN_Receive3/1 -> CAN Unpack3/1
  CAN_Receive2/1 -> CAN Unpack2/1
  Bus Creator/1 -> Bus Creator6/1  "vedio_obj_0"
  Bus Creator1/1 -> Bus Creator6/2  "vedio_obj_1"
  Bus Creator2/1 -> Bus Creator6/3  "vedio_obj_2"
  Bus Creator3/1 -> Bus Creator6/4  "vedio_obj_3"
  Bus Creator4/1 -> Bus Creator6/5  "vedio_obj_4"
  Bus Creator5/1 -> Bus Creator6/6  "vedio_obj_5"
  CAN Unpack/3 -> Data Type Conversion43/1  "CIPV_ID"
  CAN Unpack1/1 -> Data Type Conversion4/1
  CAN Unpack1/2 -> Data Type Conversion1/1
  CAN Unpack1/3 -> Data Type Conversion2/1
  CAN Unpack1/4 -> Data Type Conversion3/1
  CAN Unpack1/5 -> Data Type Conversion5/1
  CAN Unpack1/6 -> Data Type Conversion6/1
  CAN Unpack1/7 -> Data Type Conversion7/1
  CAN_Receive1/1 -> CAN Unpack1/1
  CAN Unpack2/1 -> Data Type Conversion8/1
  CAN Unpack2/2 -> Data Type Conversion9/1
  CAN Unpack2/3 -> Data Type Conversion10/1
  CAN Unpack2/4 -> Data Type Conversion11/1
  CAN Unpack2/5 -> Data Type Conversion12/1
  CAN Unpack2/6 -> Data Type Conversion13/1
  CAN Unpack2/7 -> Data Type Conversion14/1
  CAN Unpack3/1 -> Data Type Conversion15/1
  CAN Unpack3/2 -> Data Type Conversion16/1
  CAN Unpack3/3 -> Data Type Conversion17/1
  CAN Unpack3/4 -> Data Type Conversion18/1
  CAN Unpack3/5 -> Data Type Conversion19/1
  CAN Unpack3/6 -> Data Type Conversion20/1
  CAN Unpack3/7 -> Data Type Conversion21/1
  CAN Unpack4/1 -> Data Type Conversion22/1
  CAN Unpack4/2 -> Data Type Conversion23/1
  CAN Unpack4/3 -> Data Type Conversion24/1
  CAN Unpack4/4 -> Data Type Conversion25/1
  CAN Unpack4/5 -> Data Type Conversion26/1
  CAN Unpack4/6 -> Data Type Conversion27/1
  CAN Unpack4/7 -> Data Type Conversion28/1
  CAN Unpack5/1 -> Data Type Conversion29/1
  CAN Unpack5/2 -> Data Type Conversion30/1
  CAN Unpack5/3 -> Data Type Conversion31/1
  CAN Unpack5/4 -> Data Type Conversion32/1
  CAN Unpack5/5 -> Data Type Conversion33/1
  CAN Unpack5/6 -> Data Type Conversion34/1
  CAN Unpack5/7 -> Data Type Conversion35/1
  CAN Unpack6/1 -> Data Type Conversion36/1
  CAN Unpack6/2 -> Data Type Conversion37/1
  CAN Unpack6/3 -> Data Type Conversion38/1
  CAN Unpack6/4 -> Data Type Conversion39/1
  CAN Unpack6/5 -> Data Type Conversion40/1
  CAN Unpack6/6 -> Data Type Conversion41/1
  CAN Unpack6/7 -> Data Type Conversion42/1

== system D53_LKA_Software/SignalBusCreator/DTC_Indicator ==
  Bus Creator11 : BusCreator  Inputs=2
  Constant{,2..21} (21 alike) : Constant  Value=0  OutDataTypeStr=uint8
  Mux : Mux  Inputs=16
  Mux1 : Mux  Inputs=5
  bsDTC_Indicator : Outport
  wires:
  Bus Creator11/1 -> bsDTC_Indicator/1  "bsDTC_Indicator"
  Mux/1 -> Bus Creator11/1  "LKAS_BSWDTC_Status"
  Constant/1 -> Mux/1  "CANEve_e_BusOff_PSA1CAN"
  Constant2/1 -> Mux/2  "CANEve_e_BusOff_SensorCAN"
  Constant4/1 -> Mux/4  "CANEve_e_Node_ESC_Validity"
  Constant3/1 -> Mux/3  "CANEve_e_Mute_PSA1CAN"
  Constant7/1 -> Mux/7  "CANEve_e_Node_TCU_Validity"
  Constant8/1 -> Mux/8  "CANEve_e_Node_GW_Validity"
  Constant6/1 -> Mux/6  "CANEve_e_Node_EMS_Validity"
  Constant5/1 -> Mux/5  "CANEve_e_Node_EPS_Validity"
  Constant13/1 -> Mux/13  "Reserved3"
  Constant14/1 -> Mux/14  "Reserved4"
  Constant16/1 -> Mux/16  "Reserved6"
  Constant15/1 -> Mux/15  "Reserved5"
  Constant11/1 -> Mux/11  "Reserved1"
  Constant12/1 -> Mux/12  "Reserved2"
  Constant10/1 -> Mux/10  "CANEve_e_Node_Camera_Validity"
  Constant9/1 -> Mux/9  "CANEve_e_Node_Radar_Validity"
  Constant17/1 -> Mux1/1  "ACC"
  Constant18/1 -> Mux1/2  "AEB"
  Constant19/1 -> Mux1/3  "LKA"
  Constant20/1 -> Mux1/4  "LDW"
  Constant21/1 -> Mux1/5  "TJA"
  Mux1/1 -> Bus Creator11/2  "Indicator_Status"

== system D53_LKA_Software/SignalBusCreator/EPS Signal Receive and Processing (EPSRx) ==
  note: Level: 3
  Bus Creator : BusCreator  Inputs=4
  CAN Recv : S-Function  FunctionName=CAN_Rec_P  Parameters=uint8(Module-1),uint32(ID),uint8(Frameformat-1),uint8(Newflag),uint8(FIFO),double(sampletime)  SFunctionDeploymentMode=off  EnableBusSupport=off  mask(CAN_receive){Module=CAN_1, ID=1173, Frameformat=Standard (11-bit identifier), Newflag=off, FIFO=off, sampletime=0.01}
      mask prompts: Module "CAN Port:"; ID "CAN Frame ID:"; Frameformat "CAN Frame Format:"; FIFO "Overflow flag"
      mask init:
      | maskdisplay = canrecicon(Module,ID,Frameformat,Newflag,FIFO);
      | set_param(gcb, 'MaskDisplay', maskdisplay);
      mask TypeOptions Module: CAN_0 | CAN_1 | CAN_2 | CAN_3
      mask TypeOptions Frameformat: Standard (11-bit identifier) | Extended (29-bit identifier)
      mask Display: color('blue');text(0.98,0.9,'MPC5675K','horizontalAlignment','right');color('black');text(0.5,0.6,'FlexCAN_1 Receive','horizontalAlignment','center');text(0.5,0.35,'Standard ID:1173','horizontalAlignment','center');port_label('output',1,'CAN_Msg');
  CAN Unpack : canmsglib/CAN Unpack  CANdbFile=D:\ADAS ECU-PSA1 CAN_for_HIL_20190729_10ms.dbc  MsgList=EPS_495_PSA1  MsgName=EPS_495_PSA1  MsgIDType=Standard (11-bit identifier)  MsgIdentifier=1173  MsgLength=4  SignalInfo=Power_steering_status$14$2$2$2$1$0$1$0$-Inf$Inf$#State_indicating_steering_or_not$17$1$2$2$1$0$1$0$-Inf$Inf$#State_of_EPS_for_LKA_function$18$3$2$2$1$0$1$0$-Inf$Inf$#Steering_wheel_torque$0$8$2$1$1$0$2.500000e-01$0$-32$3.150000e+01$#Torque_limitation_if_DAE_limit$16$1$2$2$1$0$1$0$-Inf$Inf$#  NSignals=5  IDPort=off  TimestampPort=off  ErrorPort=off  RemotePort=off  LengthPort=off  StatusPort=off  StartBits=str2num('[int32(14);int32(17);int32(18);int32(0);int32(16)]')  SignalSizes=str2num('[int32(2);int32(1);int32(3);int32(8);int32(1)]')  ByteOrders=str2num('[int32(2);int32(2);int32(2);int32(2);int32(2)]')  DataTypes=str2num('[int32(2);int32(2);int32(2);int32(1);int32(2)]')  MultiplexTypes=str2num('[int32(1);int32(1);int32(1);int32(1);int32(1)]')  MultiplexValues=str2num('[double(0);double(0);double(0);double(0);double(0)]')  Factors=str2num('[double(1);double(1);double(1);double(2.500000e-01);double(1)]')  Offsets=str2num('[double(0);double(0);double(0);double(0);double(0)]')  Minimums=str2num('[double(-Inf);double(-Inf);double(-Inf);double(-32);double(-Inf)]')  Maximums=str2num('[double(Inf);double(Inf);double(Inf);double(3.150000e+01);double(Inf)]')  ApplyMinMax=off
      settings: SourceProductName=Simulink Real-Time  SourceProductBaseCode=XP  DataFormat=CANdb specified signals
  Data Type Conversion : DataTypeConversion  OutDataTypeStr=uint16
  Data Type Conversion1 : DataTypeConversion  OutDataTypeStr=single
  Data Type Conversion2 : DataTypeConversion  OutDataTypeStr=uint16
  Data Type Conversion3 : DataTypeConversion  OutDataTypeStr=uint16
  EPSRx_bsEPSInfo : Outport
  wires:
  Data Type Conversion3/1 -> Bus Creator/2  "EPSRx_stHandOff"
  CAN Unpack/2 -> Data Type Conversion3/1
  CAN Unpack/3 -> Data Type Conversion/1
  CAN Unpack/4 -> Data Type Conversion1/1
  CAN Recv/1 -> CAN Unpack/1
  Data Type Conversion2/1 -> Bus Creator/1  "EPSRx_efEPSErrState"
  CAN Unpack/1 -> Data Type Conversion2/1
  Data Type Conversion1/1 -> Bus Creator/4  "EPSRx_trqSWTrq"
  Data Type Conversion/1 -> Bus Creator/3  "EPSRx_stEPSCtlState"
  Bus Creator/1 -> EPSRx_bsEPSInfo/1
